simulink library "DYN_MCI"  (Simulink 8.8)
settings: Solver=ode45  StartTime=0.0  StopTime=10.0  RelTol=1e-3  EnableMultiTasking=on
undefined symbols (not defined in the file): DYN_SC_par
settings Model: Creator=alger  LastModifiedBy=alger

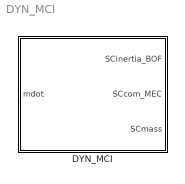
== system DYN_MCI ==
  DYN_MCI : Subsystem

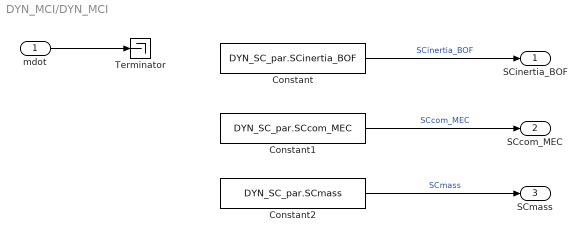
== system DYN_MCI/DYN_MCI ==
  mdot : Inport
  Constant : Constant  Value=DYN_SC_par.SCinertia_BOF
  Constant1 : Constant  Value=DYN_SC_par.SCcom_MEC
  Constant2 : Constant  Value=DYN_SC_par.SCmass  VectorParams1D=off
  Terminator : Terminator
  SCinertia_BOF : Outport
  SCcom_MEC : Outport  Port=2
  SCmass : Outport  Port=3
  wires:
  mdot/1 -> Terminator/1
  Constant/1 -> SCinertia_BOF/1  "SCinertia_BOF"
  Constant1/1 -> SCcom_MEC/1  "SCcom_MEC"
  Constant2/1 -> SCmass/1  "SCmass"
